simulink model "youhua_1226"  (R2017b)
settings: Solver=ode1  StartTime=0.0  StopTime=Inf  FixedStep=0.0002  RelTol=1e-3
PreLoadFcn:
  | initFun_4P.m
PostLoadFcn:
  | , if any(exist('dsrtsu_mdlpostloadfcn', 'file') == [2, 3, 6]), try dsrtsu_mdlpostloadfcn('Execute', bdroot); catch fprintf('Error in PostLoadFcn (dsrtsu_mdlpostloadfcn) for model "%s":\n %s\n', bdroot, lasterr); end, end,
InitFcn:
  | initFun_4P
undefined symbols (not defined in the file): CMAES_B_initial, CMAES_C_initial, CMAES_chiN_initial, CMAES_counteval_initial, CMAES_D_initial, CMAES_eigeneval_initial, CMAES_invsqrtC_initial, CMAES_pc_initial, CMAES_ps_initial, CMAES_sigma_initial, CMAES_xmean_initial
libraries: rti1202lib_adc_class1 x20, simulink x8, dsparch4 x6, rti1202serlib x4, rti1202lib_dio_class1 x4, dsextras x3, rtiemclib x2, rti1202lib_dac_class1 x1, rtitasklib x1
(part 1 of 6)
Description:
  | Standard RTI1202 template.
  | Supported MATLAB version:  R2017b.
settings Model: Tag=RTI1202  DSRTSU_INTERNAL_RTI_VER=510  DSRTSU_INTERNAL_RTI_TYPE=rti1202  RTICANMMDATA=struct('GeneralSetupData',struct('modelroot','E:\liuhang\success1226','generalsettings',struct('filesettings',struct('destfolder',struct('Name','RTICANMM_FILES','Check',1),'buildfolder',struct('Name','.','Check',1),'AbsDestfolder',struct('Name','E:\liuhang\success1226\RTICANMM_FILES'),'AbsBuildfolder',struct('Name','E:\liuhang\success1226'))),'options',struct('addpaths',1,'rmpaths',1,'addtrcexclusion',logical(1),'cannavigator',struct('checkmonitoring',0),'show_usrtrc',0,'use_usrtrc',0),'advanced',struct('options',[1 1 1 1 1 1 1 1 1 1 1 1 1 1 1 1 1 1 1 1 1 1 1 1 1 1 1 1 1 1 1 1 1 1 1 1 1 1 1 1 1 1 1 1 1 1 1 1 1 1 1 1 1 1 1 1 1 1 1 1 1 1 1 1 1 1 1 1 1 1 1 1 1 1 1 1 1 1 1 1 1 1 1 1 1 1 1 1 1 1 1 1 1 1 1 1 1 1 1 1]),'MPSetup',{{}},'modelname','youhua_1226','block','youhua_1226'))  DSRTSU_INTERNAL_RTIFLEXRAYCONFIG=110  DSRTSU_INTERNAL_RTIFPGA=110  Creator=224  LastModifiedBy=224
settings OptimizationCC: BlockReduction=off  OptimizeBlockIOStorage=off  BufferReuse=off  GlobalBufferReuse=off  ExpressionFolding=off  LocalBlockOutputs=off
settings HardwareCC: ProdBitPerPointer=32  ProdBitPerSizeT=32  ProdBitPerPtrDiffT=32  ProdLargestAtomicInteger=Integer  ProdEndianess=BigEndian  ProdWordSize=32  ProdHWDeviceType=Custom Processor->Custom  TargetIntDivRoundTo=Zero  TargetEndianess=BigEndian  TargetHWDeviceType=Custom Processor->Custom
settings SFSimCC: MATLABDynamicMemAlloc=off
settings RTWCC: SystemTargetFile=rti1202.tlc  MakeCommand=make_rti  TemplateMakefile=rti1202.tmf  Description=dSPACE DS1202 Hardware Platform
settings CodeAppCC: StateflowObjectComments=on
settings STFCustomTargetCC: ParMdlRefBuildCompliant=on  GRTInterface=off  SystemTargetFile=rti1202.tlc
settings GRTTargetCC: TargetLangStandard=C89/C90 (ANSI)  CompOptLevelCompliant=off  ConcurrentExecutionCompliant=off  CombineOutputUpdateFcns=off  MatFileLogging=off  CPPClassGenCompliant=off  UseToolchainInfoCompliant=off
settings ConfigComp: CovMetricSettings=dswe

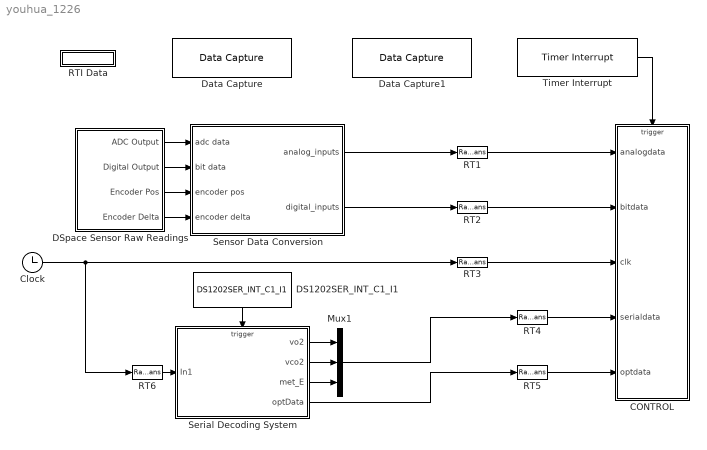
== system youhua_1226 ==
  CONTROL : Subsystem
  Clock : Clock
  DS1202SER_INT_C1_I1 : rti1202serlib/DS1202SER_INT_C1_I1  Reserved1=[]  Reserved2=[]  Reserved3=[]  Reserved4=[]  DSProperties=struct('RTI',struct('IOBoardType',{{'DS1202','SER'}},'SlaveProcessor','NONE','Version',uint32(3),'BlockType',struct('isSLSource',uint8(1),'isSLSink',uint8(0),'isHWSource',uint8(0),'isHWSink',uint8(0),'isSetup',uint8(0),'isInline',uint8(1),'isNonInline',uint8(0),'isInterrupt',uint8(1),'isChannelwise',uint8(1)),'UnitType','GENSER','Identifier','SERINT','DialogType','ML','BlockSet','NONE','RelationId',struct('TH',struct('BlockId','HWINT'))))  RTIBlockInterface=struct('BlockDisplay',{{['DS1202 SER Interrupt\n Channel 1\nReceive Interrupt'],'center'}},'BlockName',struct('Token',{{'DS1202SER_INT_C','_I'}},'BlockParam',{{'ChannelNo','IntType'}}),'OutputPortsWidth',int32(1),'OutputPortsActive',1,'OutputPortsName',{{[' ']}},'IconTransparency','off','ParameterTunableNames',{{}},'InitLevel',3,'DialogFcn','guigenserserint','MaskDescription',['To make the interrupts of the UART serial interface available as trigger source.'],'FunctionCall',uint32(0),'Options',{{'SS_OPTION_FORCE_NONINLINED_FCNCALL','SS_OPTION_ASYNCHRONOUS_INTERRUPT'}})  RTIBlockParameters=struct('ThIntNo',{{'UART_EVENTS','OFF',[]}},'ThSubIntNo',{{0,'ON',[0 4]}},'ThSrcSgnName',{{['UART Ch1 RX SW FIFO interrupt'],'OFF',[]}},'TLCFileName',{{'rti_hwinterrupt','OFF',[]}},'BoardNo',{{1,'ON',[1 1]}},'ChannelNo',{{1,'ON',[1 2]}},'ChannelNumOf',{{2,'OFF',[]}},'ThBlk',{{['struct(''blkh'',''youhua_1226/DS1202SER_INT_C1_I1'',''srcId'',''UART_EVENTS_CH1_INT0'',''srcSgnId'',''UART_EVENTS_CH1_INT0'',''intervalTmrBlockId'',[],''srcSgnName'',[''UART Ch1 RX SW FIFO interrupt''],''srcCpuId'','''',''isSrcCpu'',1,''isTargetCpu'',1,''srcOnMasterCpu'',1,''boardType'','''',''boardTypeNo'','''',''boardNo'',1,''intNo'',''UART_EVENTS'',''subIntNo'',0,''period'',0,''entryPoint'',''rti_UART_EVENTS_CH1_INT0'',''blockName'',''DS1202SER_INT_C1_I1'',''taskNameDisplayExt'','''',''taskType'',''HWINT'',''groupId'',''SERINT'',''hookFcn'',''NULL'',''isTimerTaskSrc'',0,''service'','''',''mpBlkId'','''',''taskPriorityPreConfig'',''none'',''taskPriority'',-1,''taskSortWeighting'',[],''taskSchedulingPolicy'',''FCFS'',''taskOvrPreConfig'',''none'',''taskOvrStrategy'',1,''taskOvrQueueSize'',1,''taskVisibility'',''on'',''taskGroupId'','''',''taskGroupDisplayOrder'',[],''serviceDynamicGen'',0,''disableCodeGen'',0,''boardBase'',''IOLIB_SPEC_INT_UART(1)'',''noBoardBase'','''')'],'OFF',[]}},'IntType',{{1,'ON',[1 4]}},'ReceiveIntLevelFifo',{{1,'OFF',[]}},'IntTypeMacro',{{'DSSER_TRIGGER_LEVEL_SUBINT_MASK','OFF',[]}},'FifoSizeDefault',{{64,'OFF',[]}})  RTISFcnParameters=struct('BoardNo','double','ChannelNo','double','ThIntNo','double','ThSubIntNo','double','ThBlk','struct','IntType','double','ReceiveIntLevelFifo','double','TLCFileName','char','IntTypeMacro','char')  RTIBlockParaDefault=struct('ThIntNo',1,'ThSubIntNo',0,'ThSrcSgnName',['RX SW FIFO interrupt'],'TLCFileName','rti_hwinterrupt','BoardNo',1,'ChannelNo',1,'ChannelNumOf',2,'ThBlk',['struct(''srcSgnId'', '''')'],'IntType',1,'ReceiveIntLevelFifo',1,'IntTypeMacro','DSSER_TRIGGER_LEVEL_SUBINT_MASK','FifoSizeDefault',64)
  DSpace Sensor Raw Readings : Subsystem
  Data Capture : dsextras/Data Capture  ServiceNumber=2  ServiceName=BaseSampleRate  SampleTime=-1  XAxisLabelMode=off  XAxisLabel=sec  XAxisIncrement=1  TLCFileName=rti_data_capture  XAxisUnit=[]  IncrementSetting=[]  CustomSampleTime=[]  Reserved1=[]  Reserved2=[]  Reserved3=[]  Reserved4=[]  DSProperties=struct('RTI',struct('Version',uint32(3),'BlockType',struct('isSLSource',uint8(0),'isSLSink',uint8(0),'isHWSource',uint8(0),'isHWSink',uint8(0),'isSetup',uint8(0),'isInline',uint8(1),'isNonInline',uint8(0),'isInterrupt',uint8(0),'isChannelwise',uint8(0)),'IOBoardType','EXTRAS','UnitType','DATACAP','Identifier','DATACAP','DialogType','SL','BlockSet','NONE','SlaveProcessor','NONE'))  RTIBlockInterface=struct('OutputPortsActive',0,'OutputPortsWidth',int32(0),'InitLevel',2,'BlockDisplay',{{['Host Service #2\nBaseSampleRate'],'center'}},'BlockName',struct('Token',{{['Data Capture']}}),'MaskDescription',['Places the host service code for ControlDesk in a specific task.'],'IconTransparency','off','SampleTime',{{-1}})  RTIBlockParameters=struct('ServiceNumber',{{2,'OFF',[]}},'ServiceName',{{'BaseSampleRate','OFF',[]}},'SampleTime',{{-1,'OFF',[]}},'XAxisLabelMode',{{logical(0),'OFF',[]}},'XAxisLabel',{{'sec','OFF',[]}},'XAxisIncrement',{{1,'OFF',[]}},'TLCFileName',{{'rti_data_capture','OFF',[]}})  RTISFcnParameters=struct('ServiceNumber','double','ServiceName','char','SampleTime','double','XAxisLabelMode','double','XAxisLabel','char','XAxisIncrement','double','TLCFileName','char')  RTIBlockParaDefault=struct('ServiceNumber',1,'ServiceName','<ServiceName>','SampleTime',-1,'XAxisLabelMode',0,'XAxisLabel','sec','XAxisIncrement',1,'TLCFileName','rti_data_capture')
  Data Capture1 : dsextras/Data Capture  ServiceNumber=3  ServiceName=50Hz  SampleTime=0.02  XAxisLabelMode=off  XAxisLabel=sec  XAxisIncrement=1  TLCFileName=rti_data_capture  XAxisUnit=[]  IncrementSetting=[]  CustomSampleTime=[]  Reserved1=[]  Reserved2=[]  Reserved3=[]  Reserved4=[]  DSProperties=struct('RTI',struct('Version',uint32(3),'BlockType',struct('isSLSource',uint8(0),'isSLSink',uint8(0),'isHWSource',uint8(0),'isHWSink',uint8(0),'isSetup',uint8(0),'isInline',uint8(1),'isNonInline',uint8(0),'isInterrupt',uint8(0),'isChannelwise',uint8(0)),'IOBoardType','EXTRAS','UnitType','DATACAP','Identifier','DATACAP','DialogType','SL','BlockSet','NONE','SlaveProcessor','NONE'))  RTIBlockInterface=struct('OutputPortsActive',0,'OutputPortsWidth',int32(0),'InitLevel',2,'BlockDisplay',{{['Host Service #3\n50Hz'],'center'}},'BlockName',struct('Token',{{['Data Capture']}}),'MaskDescription',['Places the host service code for ControlDesk in a specific task.'],'IconTransparency','off','SampleTime',{{0.02}})  RTIBlockParameters=struct('ServiceNumber',{{3,'OFF',[]}},'ServiceName',{{'50Hz','OFF',[]}},'SampleTime',{{0.02,'OFF',[]}},'XAxisLabelMode',{{logical(0),'OFF',[]}},'XAxisLabel',{{'sec','OFF',[]}},'XAxisIncrement',{{1,'OFF',[]}},'TLCFileName',{{'rti_data_capture','OFF',[]}})  RTISFcnParameters=struct('ServiceNumber','double','ServiceName','char','SampleTime','double','XAxisLabelMode','double','XAxisLabel','char','XAxisIncrement','double','TLCFileName','char')  RTIBlockParaDefault=struct('ServiceNumber',1,'ServiceName','<ServiceName>','SampleTime',-1,'XAxisLabelMode',0,'XAxisLabel','sec','XAxisIncrement',1,'TLCFileName','rti_data_capture')
  Mux1 : Mux  Inputs=3
  RT{1..6} (6 alike) : RateTransition  Deterministic=off
  RTI Data : Subsystem  Tag=struct('RTIDataServer',struct('RTIDataServerVs','2','RTIModelDescription','struct(''main'',''youhua_1226'',''sub'','''',''isMp'',0)'))  LoadFcn="if exist('rtidc'), try,  rtidc('DataHostBlockClbLoad', gcbh); catch, disp(['Warning: ''LoadFcn'' for RTI Data block failed: ' lasterr]); end, end,"  mask(RTI_DATA_HOST){}
      mask help:
      | RTI Data Block.
      | This block is used by RTI to store internal model-dependent data.
      | Please keep this block on the root level of the model. Deleting this block will result in data loss.
      |
      | NEVER DELETE OR COPY THIS BLOCK!
      settings: CopyFcn="if exist('rtidc'), try,  rtidc('DataHostBlockClbCopy', gcbh); catch, disp(['Warning: ''CopyFcn'' for RTI Data block failed: ' lasterr]); end, end,"  DeleteFcn="if exist('rtidc'), try,  rtidc('DataHostBlockClbDelete', gcbh); catch, disp(['Warning: ''DeleteFcn'' for RTI Data block failed: ' lasterr]); end, end,"  ModelCloseFcn="if exist('rtidc'), try,  rtidc('DataHostBlockClbModelClose', gcbh); catch, disp(['Warning: ''ModelCloseFcn'' for RTI Data block failed: ' lasterr]); end, end,"  PreSaveFcn="if exist('rtidc'), try,  rtidc('DataHostBlockClbPreSave', gcbh); catch, disp(['Warning: ''PreSaveFcn'' for RTI Data block failed: ' lasterr]); end, end,"  PostSaveFcn="if exist('rtidc'), try,  rtidc('DataHostBlockClbPostSave', gcbh); catch, disp(['Warning: ''PostSaveFcn'' for RTI Data block failed: ' lasterr]); end, end,"  NameChangeFcn="if exist('rtidc'), try,  rtidc('DataHostBlockClbNameChange', gcbh); catch, disp(['Warning: ''NameChangeFcn'' for RTI Data block failed: ' lasterr]); end, end,"
      mask Help:
      | RTI Data Block.
      | This block is used by RTI to store internal model-dependent data.
      | Please keep this block on the root level of the model. Deleting this block will result in data loss.
      | 
      | NEVER DELETE OR COPY THIS BLOCK!
      mask Display:
      | text(0.5, 0.5, 'RTI Data', 'HorizontalAlignment', 'center');
      | plot([1 0]);
  Sensor Data Conversion : Subsystem
  Serial Decoding System : Subsystem
  Timer Interrupt : rtitasklib/Timer Interrupt  DSProperties=struct('RTI',struct('Version',uint32(3),'BlockType',struct('isSLSource',uint8(1),'isSLSink',uint8(0),'isHWSource',uint8(0),'isHWSink',uint8(0),'isSetup',uint8(0),'isInline',uint8(1),'isNonInline',uint8(0),'isInterrupt',uint8(1),'isChannelwise',uint8(0)),'IOBoardType','INTLIB','UnitType','TMRINT','Identifier','TMRINT','DialogType','ML','BlockSet','NONE','SlaveProcessor','NONE','RelationId',struct('TH',struct('BlockId','TMRINT'))))  RTIBlockInterface=struct('OutputPortsActive',1,'OutputPortsWidth',int32(1),'FunctionCall',uint32(0),'OutputPortsName',{{[' ']}},'BlockDisplay',{{['DS1202 Board\nTimer B interrupt'],'center'}},'IconTransparency','on','InitLevel',3,'BlockName',struct('Token',{{['Timer Interrupt']}}),'DialogFcn','rtitasklibtmrintgui','SampleTime',{{-1}},'Options',{{'SS_OPTION_FORCE_NONINLINED_FCNCALL','SS_OPTION_ASYNCHRONOUS_INTERRUPT'}})  RTIBlockParameters=struct('ThPeriod',{{'0.002','OFF',[]}},'SampleTime',{{'-1','OFF',[]}},'ThTimerId',{{2,'OFF',[]}},'ThSrcSgnName',{{['Timer B interrupt'],'OFF',[]}},'ThBlk',{{['struct(''blkh'',[''youhua_1226/Timer Interrupt''],''srcId'',''TIMERB'',''srcSgnId'',''TIMERB'',''intervalTmrBlockId'',[],''srcSgnName'',[''Timer B interrupt''],''srcCpuId'','''',''isSrcCpu'',1,''isTargetCpu'',1,''srcOnMasterCpu'',1,''boardType'','''',''boardTypeNo'','''',''boardNo'',1,''intNo'',0,''subIntNo'',-1,''period'',''0.002'',''entryPoint'',''rti_TIMERB'',''blockName'',[''Timer Interrupt''],''taskNameDisplayExt'','''',''taskType'',''TMRINT'',''groupId'',''B'',''hookFcn'',''NULL'',''isTimerTaskSrc'',0,''service'',''S_PERIODIC_B'',''mpBlkId'','''',''taskPriorityPreConfig'',''none'',''taskPriority'',-1,''taskSortWeighting'',[],''taskSchedulingPolicy'',''FCFS'',''taskOvrPreConfig'',''none'',''taskOvrStrategy'',1,''taskOvrQueueSize'',1,''taskVisibility'',''on'',''taskGroupId'','''',''taskGroupDisplayOrder'',[],''serviceDynamicGen'',0,''disableCodeGen'',0,''boardBase'',''0'',''noBoardBase'','''')'],'OFF',[]}},'TLCFileName',{{'rtitasklibtmrint','OFF',[]}})  RTISFcnParameters=struct('ThBlk','struct','TLCFileName','char','SampleTime','double')  RTIBlockParaDefault=struct('ThPeriod',0.01,'SampleTime',-1,'ThTimerId',2,'ThSrcSgnName',['Timer B interrupt'],'ThBlk',['struct(''srcSgnId'', '''')'],'TLCFileName','rtitasklibtmrint')
  wires:
  RT3/1 -> CONTROL/3(clk)
  Serial Decoding System/1(vo2) -> Mux1/1
  Serial Decoding System/3(met_E) -> Mux1/3
  Mux1/1 -> RT4/1
  RT1/1 -> CONTROL/1(analogdata)
  RT4/1 -> CONTROL/4(serialdata)
  Serial Decoding System/2(vco2) -> Mux1/2
  RT5/1 -> CONTROL/5(optdata)
  DSpace Sensor Raw Readings/2(Digital Output) -> Sensor Data Conversion/2(bit data)
  Serial Decoding System/4(optData) -> RT5/1
  Clock/1 -> RT3/1, RT6/1
  DSpace Sensor Raw Readings/4(Encoder Delta) -> Sensor Data Conversion/4(encoder delta)
  Sensor Data Conversion/2(digital_inputs) -> RT2/1
  Sensor Data Conversion/1(analog_inputs) -> RT1/1
  DSpace Sensor Raw Readings/3(Encoder Pos) -> Sensor Data Conversion/3(encoder pos)
  RT2/1 -> CONTROL/2(bitdata)
  RT6/1 -> Serial Decoding System/1(In1)
  DSpace Sensor Raw Readings/1(ADC Output) -> Sensor Data Conversion/1(adc data)
  DS1202SER_INT_C1_I1/1 -> Serial Decoding System/Trigger
  Timer Interrupt/1 -> CONTROL/Trigger

== system youhua_1226/CONTROL ==
  analogdata : Inport
  bitdata : Inport  Port=2
  clk : Inport  Port=3
  serialdata : Inport  Port=4
  optdata : Inport  Port=5
  Trigger : TriggerPort  TriggerType=function-call  VariantControl=(inherit)
  Control and Display : Subsystem
  Data Capture1 : dsextras/Data Capture  ServiceNumber=1  ServiceName=500Hz  SampleTime=-1  XAxisLabelMode=off  XAxisLabel=sec  XAxisIncrement=1  TLCFileName=rti_data_capture  XAxisUnit=[]  IncrementSetting=[]  CustomSampleTime=[]  Reserved1=[]  Reserved2=[]  Reserved3=[]  Reserved4=[]  DSProperties=struct('RTI',struct('Version',uint32(3),'BlockType',struct('isSLSource',uint8(0),'isSLSink',uint8(0),'isHWSource',uint8(0),'isHWSink',uint8(0),'isSetup',uint8(0),'isInline',uint8(1),'isNonInline',uint8(0),'isInterrupt',uint8(0),'isChannelwise',uint8(0)),'IOBoardType','EXTRAS','UnitType','DATACAP','Identifier','DATACAP','DialogType','SL','BlockSet','NONE','SlaveProcessor','NONE'))  RTIBlockInterface=struct('OutputPortsActive',0,'OutputPortsWidth',int32(0),'InitLevel',2,'BlockDisplay',{{['Host Service #1\n500Hz'],'center'}},'BlockName',struct('Token',{{['Data Capture']}}),'MaskDescription',['Places the host service code for ControlDesk in a specific task.'],'IconTransparency','off','SampleTime',{{-1}})  RTIBlockParameters=struct('ServiceNumber',{{1,'OFF',[]}},'ServiceName',{{'500Hz','OFF',[]}},'SampleTime',{{-1,'OFF',[]}},'XAxisLabelMode',{{logical(0),'OFF',[]}},'XAxisLabel',{{'sec','OFF',[]}},'XAxisIncrement',{{1,'OFF',[]}},'TLCFileName',{{'rti_data_capture','OFF',[]}})  RTISFcnParameters=struct('ServiceNumber','double','ServiceName','char','SampleTime','double','XAxisLabelMode','double','XAxisLabel','char','XAxisIncrement','double','TLCFileName','char')  RTIBlockParaDefault=struct('ServiceNumber',1,'ServiceName','<ServiceName>','SampleTime',-1,'XAxisLabelMode',0,'XAxisLabel','sec','XAxisIncrement',1,'TLCFileName','rti_data_capture')
  Motor Controller : Subsystem
  wires:
  analogdata/1 -> Control and Display/1(analog sensor data)
  bitdata/1 -> Control and Display/2(bit sensor data)
  clk/1 -> Control and Display/3(clock)
  serialdata/1 -> Control and Display/4(serial)
  optdata/1 -> Control and Display/5(opt)
  Control and Display/1(commanded velocity) -> Motor Controller/1(Speed)

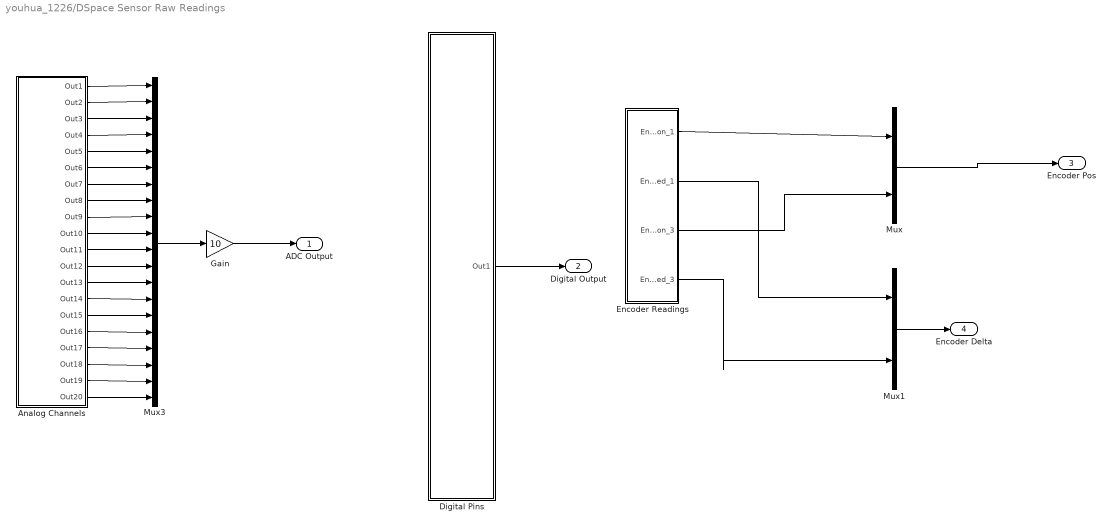
== system youhua_1226/DSpace Sensor Raw Readings ==
  Analog Channels : Subsystem
  Digital Pins : Subsystem
  Encoder Readings : Subsystem
  Gain : Gain  Gain=10
  Mux : Mux  Inputs=2
  Mux1 : Mux  Inputs=2
  Mux3 : Mux  Inputs=20
  ADC Output : Outport
  Digital Output : Outport  Port=2
  Encoder Pos : Outport  Port=3
  Encoder Delta : Outport  Port=4
  wires:
  Analog Channels/2(Out2) -> Mux3/2
  Analog Channels/3(Out3) -> Mux3/3
  Analog Channels/4(Out4) -> Mux3/4
  Analog Channels/5(Out5) -> Mux3/5
  Analog Channels/7(Out7) -> Mux3/7
  Analog Channels/8(Out8) -> Mux3/8
  Analog Channels/9(Out9) -> Mux3/9
  Analog Channels/10(Out10) -> Mux3/10
  Analog Channels/11(Out11) -> Mux3/11
  Analog Channels/12(Out12) -> Mux3/12
  Analog Channels/13(Out13) -> Mux3/13
  Analog Channels/14(Out14) -> Mux3/14
  Analog Channels/15(Out15) -> Mux3/15
  Analog Channels/16(Out16) -> Mux3/16
  Analog Channels/6(Out6) -> Mux3/6
  Analog Channels/18(Out18) -> Mux3/18
  Analog Channels/19(Out19) -> Mux3/19
  Analog Channels/20(Out20) -> Mux3/20
  Mux3/1 -> Gain/1
  Gain/1 -> ADC Output/1
  Mux/1 -> Encoder Pos/1
  Mux1/1 -> Encoder Delta/1
  Analog Channels/1(Out1) -> Mux3/1
  Analog Channels/17(Out17) -> Mux3/17
  Digital Pins/1(Out1) -> Digital Output/1
  Encoder Readings/1(Encoder_Position_1) -> Mux/1
  Encoder Readings/3(Encoder_Position_3) -> Mux/2
  Encoder Readings/2(Encoder_Speed_1) -> Mux1/1
  Encoder Readings/4(Encoder_Speed_3) -> Mux1/2

== system youhua_1226/RTI Data ==
  RTI Data Store : Subsystem  Tag="struct('private',struct('version',struct('dsVer',uint32(2),'dsVerCreation',uint32(2),'RTI',struct('ver','7.9','type','RTI1202')),'access',struct('type','Model','isPerm',1,'created',['13-Dec-2018 18:02:57'],'modified',['25-Apr-2019 21:07:37'],'location','')),'public',struct('main',struct('data',[]),'sub',struct('name',{{'youhua_1226'}},'data',{{struct('TH',struct('thTaskInfo',struct('taskType',{'TIMER','HWINT','TMRINT','SWINT','GLINT'},'tasksNumOf',{1,1,1,0,0},'srcIds',{{'TIMERA'},{'UART_EVENTS_CH1_INT0'},{'TIMERB'},{},{}},'taskNames',{{['Timer Task 1']},{'DS1202SER_INT_C1_I1'},{['Timer Interrupt']},{},{}})),'th_tc',struct('dataType',{'TASK','TASK','TASK'},'taskGroupId',{'','',''},'taskGroupList',{{},{},{}},'taskSchedulingPolicy',{'FCFS','FCFS','FCFS'},'taskType',{'TIMER','HWINT','TMRINT'},'blkh',{-1,'youhua_1226/DS1202SER_INT_C1_I1',['youhua_1226/Timer Interrupt']},'srcId',{'TIMERA','UART_EVENTS_CH1_INT0','TIMERB'},'srcSgnName',{['Timer A interrupt'],['UART Ch1 RX SW FIFO interrupt'],['Timer B interrupt']},'srcCpuName',{'','',''},'taskName',{['Timer Task 1  [0.0002] s'],'DS1202SER_INT_C1_I1',['Timer Interrupt']},'taskNameDisplayExt',{'','',''},'smplTime',{0.0002,0,0.002},'smplTimeOffs',{0,0,0},'hasFixedPriority',{0,0,0},'priority',{1,2,3},'hasFixedOvc',{0,0,0},'ovcType',{1,1,1},'ovcMax',{1,1,1}),'tc_th',struct('dataType',{'TASK','TASK','TASK'},'taskGroupId',{'','',''},'taskGroupList',{{},{},{}},'taskSchedulingPolicy',{'FCFS','FCFS','FCFS'},'taskType',{'TIMER','HWINT','TMRINT'},'blkh',{-1,'youhua_1226/DS1202SER_INT_C1_I1',['youhua_1226/Timer Interrupt']},'srcId',{'TIMERA','UART_EVENTS_CH1_INT0','TIMERB'},'srcSgnName',{['Timer A interrupt'],['UART Ch1 RX SW FIFO interrupt'],['Timer B interrupt']},'srcCpuName',{'','',''},'taskName',{['Timer Task 1  [0.0002] s'],'DS1202SER_INT_C1_I1',['Timer Interrupt']},'taskNameDisplayExt',{'','',''},'smplTime',{0.0002,0,0.002},'smplTimeOffs',{0,0,0},'hasFixedPriority',{0,0,0},'priority',{1,2,3},'hasFixedOvc',{0,0,0},'ovcType',{1,1,1},'ovcMax',{1,1,1}))}})))"  mask(RTI_DATA_STORE){}
      mask help:
      | RTI Data Store Block. This block is used by RTI to store internal model dependent data. Deleting this block will result in data loss.
      |
      | NEVER DELETE, COPY, OR MODIFY THIS BLOCK!
      mask Help:
      | RTI Data Store Block. This block is used by RTI to store internal model dependent data. Deleting this block will result in data loss.
      | 
      | NEVER DELETE, COPY, OR MODIFY THIS BLOCK!
      mask Display: text(0.5, 0.5, ' ', 'HorizontalAlignment', 'center');

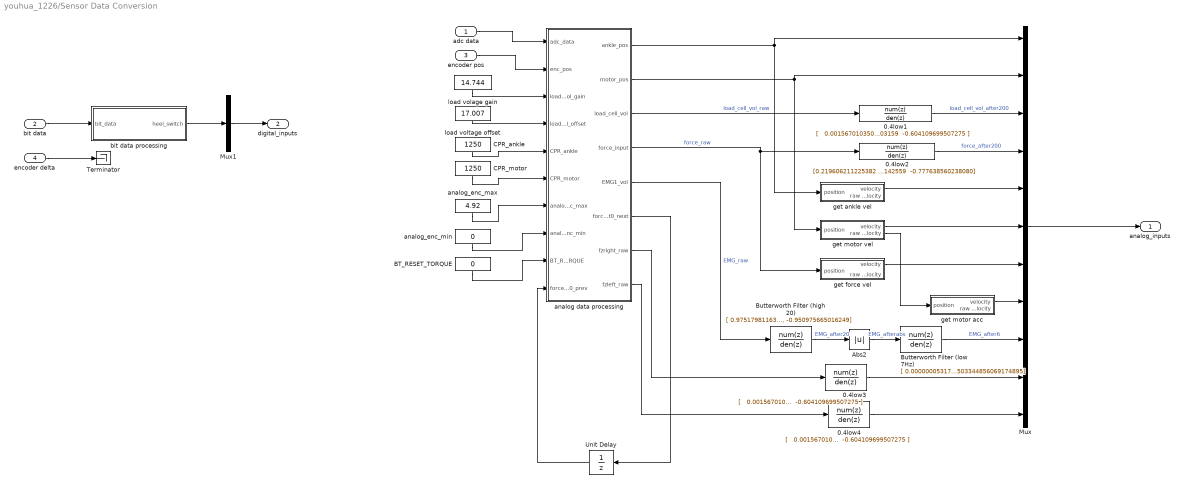
== system youhua_1226/Sensor Data Conversion ==
  adc data : Inport
  bit data : Inport  Port=2
  encoder pos : Inport  Port=3
  encoder delta : Inport  Port=4
  0.4low1 : DiscreteFilter  Numerator=|  Denominator=|
      Numerator=|
      | [   0.001567010350588   0.004701031051765   0.004701031051765   0.001567010350588
      | ]
      Denominator=|
      | [   1.000000000000000  -2.498608344691178   2.115254127003159  -0.604109699507275
      | ]
  0.4low2 : DiscreteFilter  Numerator="[0.219606211225382   0.658818633676145   0.658818633676145   0.219606211225382]*1e-3"  Denominator="[1.000000000000000  -2.748835809214676   2.528231219142559  -0.777638560238080]"
  0.4low3 : DiscreteFilter  Numerator=|  Denominator=|
      Numerator=|
      | [   0.001567010350588   0.004701031051765   0.004701031051765   0.001567010350588
      | ]
      Denominator=|
      | [   1.000000000000000  -2.498608344691178   2.115254127003159  -0.604109699507275
      | ]
  0.4low4 : DiscreteFilter  Numerator=|  Denominator=|
      Numerator=|
      | [   0.001567010350588   0.004701031051765   0.004701031051765   0.001567010350588
      | ]
      Denominator=|
      | [   1.000000000000000  -2.498608344691178   2.115254127003159  -0.604109699507275
      | ]
  Abs2 : Abs
  BT_RESET_TORQUE : Constant  Value=0
  Butterworth Filter (high 20) : DiscreteFilter  Numerator=[ 0.975179811634754, -2.92553943490426, 2.92553943490426, -0.975179811634754]  Denominator=[ 1.0, -2.94973583970635, 2.90072698835544, -0.950975665016249]
  Butterworth Filter (low 7Hz) : DiscreteFilter  Numerator=[ 0.000000053177145076244158872, 0.00000015953143522873247662, 0.00000015953143522873247662, 0.000000053177145076244158872]  Denominator=[ 1.0, -2.9849203909800881007, 2.9699542649579404596, -0.98503344856069174895]
  CPR_ankle : Constant  Value=1250
  CPR_motor : Constant  Value=1250
  Mux : Mux  Inputs=11
  Mux1 : Mux  Inputs=1
  Terminator : Terminator
  Unit Delay : UnitDelay  SampleTime=-1
  analog data processing : MATLAB Function  TreatAsAtomicUnit=on
  analog_enc_max : Constant  Value=4.92
  analog_enc_min : Constant  Value=0
  bit data processing : MATLAB Function  TreatAsAtomicUnit=on
  get ankle vel : Subsystem
  get force vel : Subsystem
  get motor acc : Subsystem
  get motor vel : Subsystem
  load volage gain : Constant  Value=14.744
  load voltage offset : Constant  Value=17.007
  analog_inputs : Outport
  digital_inputs : Outport  Port=2
  wires:
  adc data/1 -> analog data processing/1(adc_data)
  encoder delta/1 -> Terminator/1
  bit data/1 -> bit data processing/1(bit_data)
  bit data processing/1(heel_switch) -> Mux1/1
  analog data processing/1(ankle_pos) -> get ankle vel/1(position), Mux/1
  analog data processing/2(motor_pos) -> get motor vel/1(position), Mux/2
  analog data processing/4(force_input) -> get force vel/1(position), 0.4low2/1  "force_raw"
  Mux/1 -> analog_inputs/1
  Mux1/1 -> digital_inputs/1
  analog data processing/3(load_cell_vol) -> 0.4low1/1  "load_cell_vol_raw"
  load volage gain/1 -> analog data processing/3(load_vol_gain)
  load voltage offset/1 -> analog data processing/4(load_vol_offset)
  CPR_ankle/1 -> analog data processing/5(CPR_ankle)
  get ankle vel/1(velocity) -> Mux/5
  get motor vel/1(velocity) -> Mux/6
  get force vel/1(velocity) -> Mux/7
  get motor vel/2(raw velocity) -> get motor acc/1(position)
  get motor acc/1(velocity) -> Mux/8
  analog data processing/5(EMG1_vol) -> Butterworth Filter (high 20)/1  "EMG_raw"
  Butterworth Filter (low 7Hz)/1 -> Mux/9  "EMG_after6"
  Abs2/1 -> Butterworth Filter (low 7Hz)/1  "EMG_afterabs"
  Butterworth Filter (high 20)/1 -> Abs2/1  "EMG_after20"
  analog_enc_max/1 -> analog data processing/7(analog_enc_max)
  analog_enc_min/1 -> analog data processing/8(analog_enc_min)
  0.4low2/1 -> Mux/4  "force_after200"
  0.4low1/1 -> Mux/3  "load_cell_vol_after200"
  CPR_motor/1 -> analog data processing/6(CPR_motor)
  analog data processing/6(force_input0_next) -> Unit Delay/1
  Unit Delay/1 -> analog data processing/10(force_input0_prev)
  BT_RESET_TORQUE/1 -> analog data processing/9(BT_RESET_TORQUE)
  analog data processing/7(fzright_raw) -> 0.4low3/1
  analog data processing/8(fzleft_raw) -> 0.4low4/1
  0.4low3/1 -> Mux/10
  0.4low4/1 -> Mux/11
  encoder pos/1 -> analog data processing/2(enc_pos)

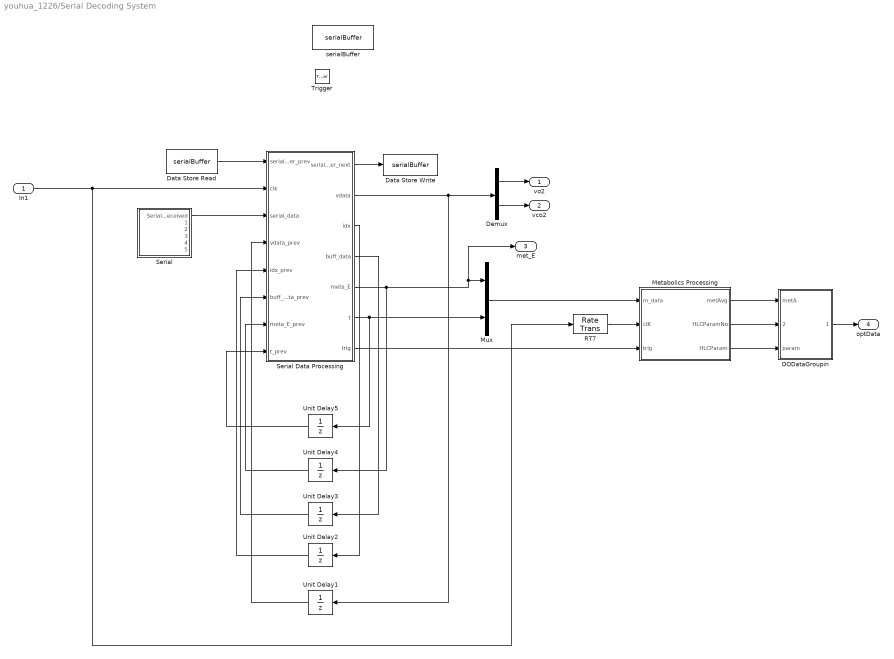
== system youhua_1226/Serial Decoding System ==
  In1 : Inport
  Trigger : TriggerPort  TriggerType=function-call  VariantControl=(inherit)
  Data Store Read : DataStoreRead  DataStoreName=serialBuffer
  Data Store Write : DataStoreWrite  DataStoreName=serialBuffer
  Demux : Demux  Outputs=2
  Metabolics Processing : Subsystem
  Mux : Mux  Inputs=2
  OODataGroupin : MATLAB Function  TreatAsAtomicUnit=on
  RT7 : RateTransition  Deterministic=off
  Serial : Subsystem
  Serial Data Processing : MATLAB Function  TreatAsAtomicUnit=on
  Unit Delay1 : UnitDelay  InitialCondition=[0;0]  SampleTime=-1
  Unit Delay2 : UnitDelay  InitialCondition=[0;0]  SampleTime=-1
  Unit Delay3 : UnitDelay  InitialCondition=[0 0 0 0 0; 0 0 0 0 0]  SampleTime=-1
  Unit Delay4 : UnitDelay  SampleTime=-1
  Unit Delay5 : UnitDelay  SampleTime=-1
  serialBuffer : DataStoreMemory  DataStoreName=serialBuffer  ReadBeforeWriteMsg=warning  WriteAfterWriteMsg=warning  WriteAfterReadMsg=warning  InitialValue=zeros(2,100)  ShowAdditionalParam=off
  vo2 : Outport
  vco2 : Outport  Port=2
  met_E : Outport  Port=3
  optData : Outport  Port=4
  wires:
  Serial/1(SerialReceived) -> Serial Data Processing/3(serial_data)
  Serial Data Processing/3(idx) -> Unit Delay2/1
  Serial Data Processing/2(vdata) -> Unit Delay1/1, Demux/1
  Serial Data Processing/4(buff_data) -> Unit Delay3/1
  Unit Delay2/1 -> Serial Data Processing/5(idx_prev)
  Unit Delay1/1 -> Serial Data Processing/4(vdata_prev)
  Unit Delay3/1 -> Serial Data Processing/6(buff_data_prev)
  Demux/2 -> vco2/1
  Demux/1 -> vo2/1
  Serial Data Processing/5(meta_E) -> Unit Delay4/1, Mux/1, met_E/1
  Unit Delay4/1 -> Serial Data Processing/7(meta_E_prev)
  Serial Data Processing/6(t) -> Unit Delay5/1, Mux/2
  Unit Delay5/1 -> Serial Data Processing/8(t_prev)
  In1/1 -> RT7/1, Serial Data Processing/2(clk)
  RT7/1 -> Metabolics Processing/2(clK)
  Metabolics Processing/1(metAvg) -> OODataGroupin/1(metA)
  Metabolics Processing/2(HLCParamNo) -> OODataGroupin/2(paramNo)
  Metabolics Processing/3(HLCParam) -> OODataGroupin/3(param)
  Mux/1 -> Metabolics Processing/1(m_data)
  Serial Data Processing/7(trig) -> Metabolics Processing/3("trig ")
  OODataGroupin/1(optdata) -> optData/1
  Serial Data Processing/1(serial_buffer_next) -> Data Store Write/1
  Data Store Read/1 -> Serial Data Processing/1(serial_buffer_prev)

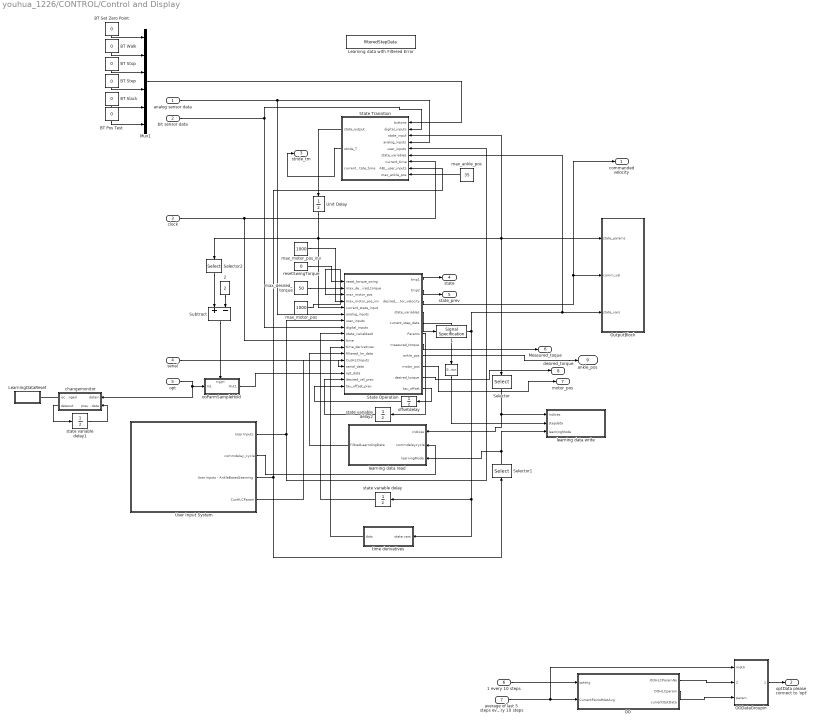
== system youhua_1226/CONTROL/Control and Display ==
  analog sensor data : Inport
  bit sensor data : Inport  Port=2
  clock : Inport  Port=3
  serial : Inport  Port=4
  opt : Inport  Port=5
  1 every 10 steps : Inport  Port=6
  average of last 5 steps every 10 steps : Inport  Port=7
  " " : SignalSpecification  Dimensions=3
  " 1" : SignalSpecification  Dimensions=52
  " Learning data with Filtered Error" : DataStoreMemory  DataStoreName=filteredStepData  ReadBeforeWriteMsg=warning  WriteAfterWriteMsg=warning  WriteAfterReadMsg=warning  InitialValue=zeros(2,450)  ShowAdditionalParam=off
  2 : Constant  Value=2
  BT Pos Test : Constant  Value=0
  BT Set Zero Point : Constant  Value=0
  BT Slack : Constant  Value=0
  BT Step : Constant  Value=0
  BT Stop : Constant  Value=0
  BT Walk : Constant  Value=0
  LearningDataReset : Subsystem  TreatAsAtomicUnit=on
  Mux1 : Mux  Inputs=6
  OO : Subsystem
  OODataGroupin : MATLAB Function  TreatAsAtomicUnit=on
  OutputBlock : Subsystem
  Selector : Selector  InputPortWidth=16  IndexOptions=Index vector (dialog)  Indices=[12 16]  OutputSizes=1
  Selector1 : Selector  InputPortWidth=3  IndexOptions=Index vector (dialog)  Indices=[3]  OutputSizes=1
  Selector2 : Selector  InputPortWidth=16  IndexOptions=Index vector (dialog)  Indices=[1]  OutputSizes=1
  State Operation : MATLAB Function  TreatAsAtomicUnit=on
  State Transition : MATLAB Function  TreatAsAtomicUnit=on
  Subtract : Sum  Inputs=+-
  Unit Delay : UnitDelay  SampleTime=-1
  User Input System : Subsystem
  changemonitor : MATLAB Function  TreatAsAtomicUnit=on
  learning data read : Subsystem
  learning data write : Subsystem
  max_ankle_pos : Constant  Value=35
  max_desired_torque : Constant  Value=50
  max_motor_pos : Constant  Value=1000
  max_motor_pos_inv : Constant  Value=1000
  offsetdelay : UnitDelay  SampleTime=-1
  ooParmSampleHold : Subsystem  TreatAsAtomicUnit=on
  resetSwingTorque : Constant  Value=0
  state variable delay : UnitDelay  InitialCondition=zeros(52,1)  SampleTime=-1
  state variable delay1 : UnitDelay  SampleTime=-1
  state variable delay2 : UnitDelay  SampleTime=-1
  "time derivatives " : Subsystem
  commanded velocity : Outport
  optData please connect to 'opt' : Outport  Port=2
  stride_tm : Outport  Port=3
  state : Outport  Port=4
  state_prev : Outport  Port=5
  Measured_toque : Outport  Port=6
  motor_pos : Outport  Port=7
  desired_torque : Outport  Port=8
  ankle_pos : Outport  Port=9
  wires:
  analog sensor data/1 -> State Transition/4(analog_inputs), State Operation/6(analog_inputs)
  State Operation/3(desired_motor_velocity) -> commanded velocity/1, OutputBlock/2(comm_vel)
  User Input System/1(User Inputs) -> State Operation/7(user_inputs), State Transition/5(user_inputs)
  BT Set Zero Point/1 -> Mux1/1
  BT Walk/1 -> Mux1/2
  BT Stop/1 -> Mux1/3
  Mux1/1 -> State Transition/1(buttons)
  BT Step/1 -> Mux1/4
  bit sensor data/1 -> State Transition/2(digital_inputs), State Operation/8(digital_inputs)
  state variable delay/1 -> State Operation/9(state_variables0)
  clock/1 -> State Transition/7(current_time), State Operation/10(time)
  BT Slack/1 -> Mux1/5
  State Transition/1(state_output) -> Unit Delay/1
  State Operation/5(current_step_data) -> " "/1
  Selector/1 -> learning data read/1(indices), learning data write/1(indices)
  Unit Delay/1 -> State Operation/5(current_state_input), State Transition/3(state_input), OutputBlock/1(state_params), Selector/1, Selector2/1
  State Operation/4(state_variables) -> " 1"/1
  " 1"/1 -> State Transition/6(state_variables), OutputBlock/3(state_vars), state variable delay/1, "time derivatives "/1(state vars)
  BT Pos Test/1 -> Mux1/6
  "time derivatives "/1(dots) -> State Operation/11(time_derivatives)
  learning data read/1(filtredLearndingData) -> State Operation/12(filtered_lrn_data)
  " "/1 -> learning data write/2(stepdata)
  User Input System/2(commdelay_cycle) -> learning data read/2(commdelaycycle)
  User Input System/3(User Inputs - AnkleBasedLearning) -> State Transition/8(ABL_user_inputs), Selector1/1
  Selector1/1 -> learning data write/3(learningMode), learning data read/3(learningMode)
  User Input System/4(CusHLCParam) -> State Operation/13(CusHLCInputs)
  serial/1 -> State Operation/14(serial_data)
  opt/1 -> changemonitor/1(datain), ooParmSampleHold/1(In1)
  ooParmSampleHold/1(Out1) -> State Operation/15(opt_data)
  changemonitor/2(dataout) -> state variable delay1/1
  state variable delay1/1 -> changemonitor/2(prev_data)
  changemonitor/1(ischanged) -> LearningDataReset/Trigger
  Selector2/1 -> Subtract/1
  2/1 -> Subtract/2
  Subtract/1 -> ooParmSampleHold/Trigger
  max_ankle_pos/1 -> State Transition/9(max_ankle_pos)
  State Operation/6(Params) -> state variable delay2/1
  state variable delay2/1 -> State Operation/16(desired_vel_prev)
  resetSwingTorque/1 -> State Operation/1(reset_torque_swing)
  State Operation/11(tau_offset) -> offsetdelay/1
  offsetdelay/1 -> State Operation/17(tau_offset_prev)
  OO/1(OOHLCParamNo) -> OODataGroupin/2(paramNo)
  1 every 10 steps/1 -> OO/1(opttrig)
  OODataGroupin/1(optdata) -> optData please connect to 'opt'/1
  average of last 5 steps every 10 steps/1 -> OODataGroupin/1(metA), OO/2(CurrentPeirodMetAvg)
  OO/2(OOHLCparam) -> OODataGroupin/3(param)
  State Transition/2(stride_T) -> stride_tm/1
  State Operation/1(tmp1) -> state/1
  State Operation/2(tmp2) -> state_prev/1
  State Operation/7(measured_torque) -> Measured_toque/1
  State Operation/9(motor_pos) -> motor_pos/1
  State Operation/10(desired_torque) -> desired_torque/1
  max_desired_torque/1 -> State Operation/2(max_desired_torque)
  max_motor_pos/1 -> State Operation/3(max_motor_pos)
  max_motor_pos_inv/1 -> State Operation/4(max_motor_pos_inv)
  State Operation/8(ankle_pos) -> ankle_pos/1

== system youhua_1226/CONTROL/Motor Controller ==
  Speed : Inport
  DAC_CLASS1_BL1 : rti1202lib_dac_class1/DAC_CLASS1_BL1  DSProperties=struct('RTI',struct('Version',uint32(2),'BlockType',struct('isSLSource',uint8(0),'isSLSink',uint8(1),'isHWSource',uint8(0),'isHWSink',uint8(1),'isSetup',uint8(0),'isInline',uint8(1),'isNonInline',uint8(0),'isInterrupt',uint8(0),'isChannelwise',uint8(1)),'IOBoardType',{{'DS120X','STD','DACC1'}},'UnitType','DAC','Identifier','DAC','DialogType','ML','BlockSet','NONE','SlaveProcessor','NONE'))  RTIBlockInterface=struct('InputPortsActive',1,'InputPortsWidth',int32(1),'InputPortsDataType',{{'SS_DOUBLE'}},'InputPortsName',{{['DAC 16']}},'DialogFcn','rti120xstddacc1dacgui','InitLevel',3,'IconTransparency','on','BlockDisplay',{{['DAC CL1\nChannel: 16'],'center'}},'BlockName',struct('Token',{{'DAC_CLASS1_BL1'}}))  RTIBlockParameters=struct('ChannelNo',{{16,'OFF',[]}},'ChannelNumOf',{{1,'OFF',[]}},'InitialValue1',{{'0','OFF',[-10 10]}},'InitialValue2',{{'0','OFF',[-10 10]}},'InitialValue3',{{'0','OFF',[-10 10]}},'InitialValue4',{{'0','OFF',[-10 10]}},'InitialValue5',{{'0','OFF',[-10 10]}},'InitialValue6',{{'0','OFF',[-10 10]}},'InitialValue7',{{'0','OFF',[-10 10]}},'InitialValue8',{{'0','OFF',[-10 10]}},'InitialValue9',{{'0','OFF',[-10 10]}},'InitialValue10',{{'0','OFF',[-10 10]}},'InitialValue11',{{'0','OFF',[-10 10]}},'InitialValue12',{{'0','OFF',[-10 10]}},'InitialValue13',{{'0','OFF',[-10 10]}},'InitialValue14',{{'0','OFF',[-10 10]}},'InitialValue15',{{'0','OFF',[-10 10]}},'InitialValue16',{{'0','OFF',[-10 10]}},'OutputMode',{{ones(1,16),'OFF',[1 2]}},'TermValue1',{{'0','OFF',[-10 10]}},'TermValue2',{{'0','OFF',[-10 10]}},'TermValue3',{{'0','OFF',[-10 10]}},'TermValue4',{{'0','OFF',[-10 10]}},'TermValue5',{{'0','OFF',[-10 10]}},'TermValue6',{{'0','OFF',[-10 10]}},'TermValue7',{{'0','OFF',[-10 10]}},'TermValue8',{{'0','OFF',[-10 10]}},'TermValue9',{{'0','OFF',[-10 10]}},'TermValue10',{{'0','OFF',[-10 10]}},'TermValue11',{{'0','OFF',[-10 10]}},'TermValue12',{{'0','OFF',[-10 10]}},'TermValue13',{{'0','OFF',[-10 10]}},'TermValue14',{{'0','OFF',[-10 10]}},'TermValue15',{{'0','OFF',[-10 10]}},'TermValue16',{{'0','OFF',[-10 10]}},'EnableTermMode',{{0,'OFF',[0 1]}},'TLCFileName',{{'rti120xdac_c1_dac','OFF',[]}},'InitialValueBuildCheck1',{{0,'OFF',[]}},'InitialValueBuildCheck2',{{0,'OFF',[]}},'InitialValueBuildCheck3',{{0,'OFF',[]}},'InitialValueBuildCheck4',{{0,'OFF',[]}},'InitialValueBuildCheck5',{{0,'OFF',[]}},'InitialValueBuildCheck6',{{0,'OFF',[]}},'InitialValueBuildCheck7',{{0,'OFF',[]}},'InitialValueBuildCheck8',{{0,'OFF',[]}},'InitialValueBuildCheck9',{{0,'OFF',[]}},'InitialValueBuildCheck10',{{0,'OFF',[]}},'InitialValueBuildCheck11',{{0,'OFF',[]}},'InitialValueBuildCheck12',{{0,'OFF',[]}},'InitialValueBuildCheck13',{{0,'OFF',[]}},'InitialValueBuildCheck14',{{0,'OFF',[]}},'InitialValueBuildCheck15',{{0,'OFF',[]}},'InitialValueBuildCheck16',{{1,'OFF',[]}},'TermValueBuildCheck1',{{0,'OFF',[]}},'TermValueBuildCheck2',{{0,'OFF',[]}},'TermValueBuildCheck3',{{0,'OFF',[]}},'TermValueBuildCheck4',{{0,'OFF',[]}},'TermValueBuildCheck5',{{0,'OFF',[]}},'TermValueBuildCheck6',{{0,'OFF',[]}},'TermValueBuildCheck7',{{0,'OFF',[]}},'TermValueBuildCheck8',{{0,'OFF',[]}},'TermValueBuildCheck9',{{0,'OFF',[]}},'TermValueBuildCheck10',{{0,'OFF',[]}},'TermValueBuildCheck11',{{0,'OFF',[]}},'TermValueBuildCheck12',{{0,'OFF',[]}},'TermValueBuildCheck13',{{0,'OFF',[]}},'TermValueBuildCheck14',{{0,'OFF',[]}},'TermValueBuildCheck15',{{0,'OFF',[]}},'TermValueBuildCheck16',{{0,'OFF',[]}})  RTISFcnParameters=struct('ChannelNo','int16','ChannelNumOf','int16','InitialValue1','double','InitialValue2','double','InitialValue3','double','InitialValue4','double','InitialValue5','double','InitialValue6','double','InitialValue7','double','InitialValue8','double','InitialValue9','double','InitialValue10','double','InitialValue11','double','InitialValue12','double','InitialValue13','double','InitialValue14','double','InitialValue15','double','InitialValue16','double','OutputMode','int16','TermValue1','double','TermValue2','double','TermValue3','double','TermValue4','double','TermValue5','double','TermValue6','double','TermValue7','double','TermValue8','double','TermValue9','double','TermValue10','double','TermValue11','double','TermValue12','double','TermValue13','double','TermValue14','double','TermValue15','double','TermValue16','double','EnableTermMode','int16','TLCFileName','char')  RTIBlockParaDefault=struct('ChannelNo',1,'ChannelNumOf',1,'InitialValue1',0,'InitialValue2',0,'InitialValue3',0,'InitialValue4',0,'InitialValue5',0,'InitialValue6',0,'InitialValue7',0,'InitialValue8',0,'InitialValue9',0,'InitialValue10',0,'InitialValue11',0,'InitialValue12',0,'InitialValue13',0,'InitialValue14',0,'InitialValue15',0,'InitialValue16',0,'OutputMode',ones(1,16),'TermValue1',0,'TermValue2',0,'TermValue3',0,'TermValue4',0,'TermValue5',0,'TermValue6',0,'TermValue7',0,'TermValue8',0,'TermValue9',0,'TermValue10',0,'TermValue11',0,'TermValue12',0,'TermValue13',0,'TermValue14',0,'TermValue15',0,'TermValue16',0,'EnableTermMode',0,'TLCFileName','rti120xdac_c1_dac','InitialValueBuildCheck1',0,'InitialValueBuildCheck2',0,'InitialValueBuildCheck3',0,'InitialValueBuildCheck4',0,'InitialValueBuildCheck5',0,'InitialValueBuildCheck6',0,'InitialValueBuildCheck7',0,'InitialValueBuildCheck8',0,'InitialValueBuildCheck9',0,'InitialValueBuildCheck10',0,'InitialValueBuildCheck11',0,'InitialValueBuildCheck12',0,'InitialValueBuildCheck13',0,'InitialValueBuildCheck14',0,'InitialValueBuildCheck15',0,'InitialValueBuildCheck16',0,'TermValueBuildCheck1',0,'TermValueBuildCheck2',0,'TermValueBuildCheck3',0,'TermValueBuildCheck4',0,'TermValueBuildCheck5',0,'TermValueBuildCheck6',0,'TermValueBuildCheck7',0,'TermValueBuildCheck8',0,'TermValueBuildCheck9',0,'TermValueBuildCheck10',0,'TermValueBuildCheck11',0,'TermValueBuildCheck12',0,'TermValueBuildCheck13',0,'TermValueBuildCheck14',0,'TermValueBuildCheck15',0,'TermValueBuildCheck16',0)
  Gain1 : Gain  Gain=1/20
  Gain2 : Gain  Gain=1/360
  wires:
  Gain2/1 -> Gain1/1
  Gain1/1 -> DAC_CLASS1_BL1/1
  Speed/1 -> Gain2/1
